simulink subsystem "PvtSubSys_PLAN_AP"  (R2020b)
settings: Solver=VariableStepAuto  StartTime=0.0  StopTime=10.0  RelTol=1e-3
undefined symbols (not defined in the file or in its folder): C_LongCtrl_0_Single, C_LongCtrl_0_Uint8, C_LongCtrl_Mph2Kph, magnitude, P_LongCtrl_accelTargAbsThrd, P_LongCtrl_AddVelAccelChange, P_LongCtrl_AddVelAccelThrd, P_LongCtrl_AddVelDistDesThrd, P_LongCtrl_AddVelEnable, P_LongCtrl_AddVelRefMsThrd, P_LongCtrl_ALaLowerChar, P_LongCtrl_ALaUpperCharEco, P_LongCtrl_ALaUpperCharNormal, P_LongCtrl_ALaUpperCharSport, P_LongCtrl_ALCAccLimitByDangerXAxis, P_LongCtrl_ALCAccLimitByDangerYAxis, P_LongCtrl_ALvAcceleLowerChar, P_LongCtrl_ALvAcceleUpperCharEco, P_LongCtrl_ALvAcceleUpperCharNormal, P_LongCtrl_ALvAcceleUpperCharSport, P_LongCtrl_CCaccelCCNeg2PosJerk, P_LongCtrl_CCaccelCCPosJerk, P_LongCtrl_CCaccelLowerIsLaneChange, P_LongCtrl_CCaccelMaxLCActive, P_LongCtrl_CCaccelMinECOAL, P_LongCtrl_CCaccelMinFastDecel, P_LongCtrl_CCaccelMinNoFastDecel, P_LongCtrl_CCaccelMinNormAL, P_LongCtrl_CCaccelMinSportAL, P_LongCtrl_CCaccelUpperCC, P_LongCtrl_CCaccelUpperCCSafeStop, P_LongCtrl_CCaMinNegAcceleLowerBand, P_LongCtrl_CCaMinNegAcceleUpperBand, P_LongCtrl_CCaMinPosAcceleLowerBand, P_LongCtrl_CCaMinPosAcceleUpperBand, P_LongCtrl_CCbECO, P_LongCtrl_CCbNorm, P_LongCtrl_CCbSport, P_LongCtrl_CCcoefESPSpd2IPSpd1, P_LongCtrl_CCcoefESPSpd2IPSpd2, P_LongCtrl_CCdecelCCJerk, P_LongCtrl_CCdecelCCJerkNegVLCInternalAcc, P_LongCtrl_CCfacNegAcceleLowerBand, P_LongCtrl_CCfacNegAcceleUpperBand, P_LongCtrl_CCfacPosAcceleLowerBand, P_LongCtrl_CCfacPosAcceleUpperBand, P_LongCtrl_CCkECO, P_LongCtrl_CCkNorm, P_LongCtrl_CCkSport, P_LongCtrl_CCLCIncSetSpdAdd, P_LongCtrl_CCLCIncSetSpdAddCntStartValue, P_LongCtrl_CCResumeDelayDeltaVel, P_LongCtrl_CCtAcceleTimeNeg, P_LongCtrl_CCtAcceleTimeNegCorrXAxis, P_LongCtrl_CCtAcceleTimeNegCorrYAxis, P_LongCtrl_CCtAcceleTimePos, P_LongCtrl_CCtAcceleTimePosCorrXAxis, P_LongCtrl_CCtAcceleTimePosCorrYAxis, P_LongCtrl_CCtStepVelPlan, P_LongCtrl_CCtTotVelPlan ... (+150)
libraries: simulink x62, TrueDurationTime x1
(part 2 of 7)

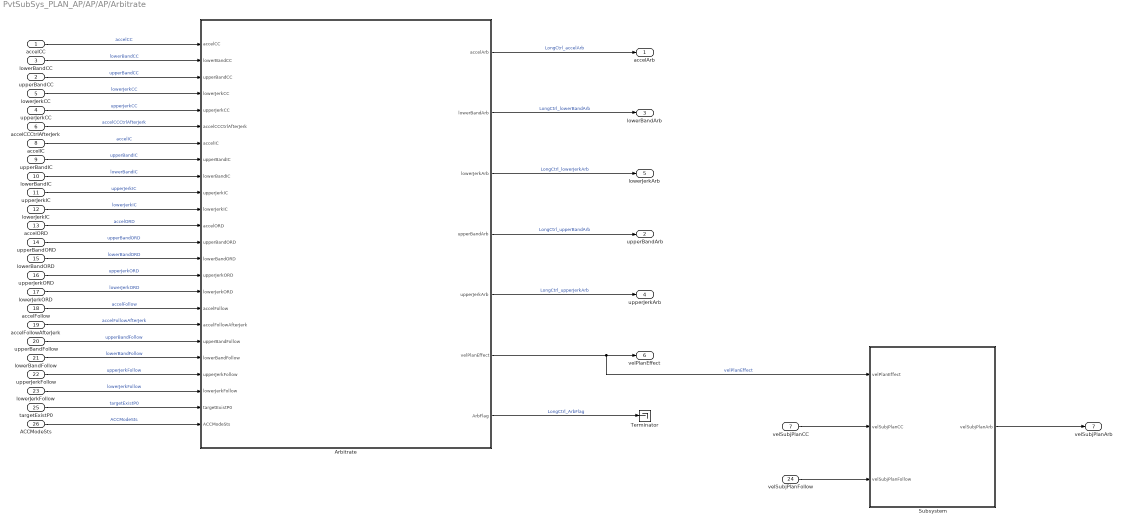
== system PvtSubSys_PLAN_AP/AP/AP/Arbitrate ==
  accelCC : Inport  OutDataTypeStr=single
  upperBandCC : Inport  Port=2  OutDataTypeStr=single
  lowerBandCC : Inport  Port=3  OutDataTypeStr=single
  upperJerkCC : Inport  Port=4  OutDataTypeStr=single
  lowerJerkCC : Inport  Port=5  OutDataTypeStr=single
  accelCCCtrlAfterJerk : Inport  Port=6  OutDataTypeStr=single
  velSubjPlanCC : Inport  Port=7
  accelIC : Inport  Port=8  OutDataTypeStr=single
  upperBandIC : Inport  Port=9  OutDataTypeStr=single
  lowerBandIC : Inport  Port=10  OutDataTypeStr=single
  upperJerkIC : Inport  Port=11  OutDataTypeStr=single
  lowerJerkIC : Inport  Port=12  OutDataTypeStr=single
  accelORD : Inport  Port=13
  upperBandORD : Inport  Port=14
  lowerBandORD : Inport  Port=15
  upperJerkORD : Inport  Port=16
  lowerJerkORD : Inport  Port=17
  accelFollow : Inport  Port=18  OutDataTypeStr=single
  accelFollowAfterJerk : Inport  Port=19
  upperBandFollow : Inport  Port=20  OutDataTypeStr=single
  lowerBandFollow : Inport  Port=21  OutDataTypeStr=single
  upperJerkFollow : Inport  Port=22  OutDataTypeStr=single
  lowerJerkFollow : Inport  Port=23  OutDataTypeStr=single
  velSubjPlanFollow : Inport  Port=24
  targetExistP0 : Inport  Port=25  OutDataTypeStr=boolean
  ACCModeSts : Inport  Port=26  OutDataTypeStr=uint8
  Arbitrate : Stateflow chart  TreatAsAtomicUnit=on
  Subsystem : Subsystem
  Terminator : Terminator
  accelArb : Outport  OutDataTypeStr=single
  " upperBandArb" : Outport  Port=2  OutDataTypeStr=single
  " lowerBandArb" : Outport  Port=3  OutDataTypeStr=single
  " upperJerkArb" : Outport  Port=4  OutDataTypeStr=single
  lowerJerkArb : Outport  Port=5  OutDataTypeStr=single
  velPlanEffect : Outport  Port=6  OutDataTypeStr=uint8
  velSubjPlanArb : Outport  Port=7  OutDataTypeStr=single
  wires:
  Arbitrate/7(ArbFlag) -> Terminator/1  "LongCtrl_ArbFlag"
  lowerJerkIC/1 -> Arbitrate/11(lowerJerkIC)  "lowerJerkIC"
  upperJerkIC/1 -> Arbitrate/10(upperJerkIC)  "upperJerkIC"
  lowerBandIC/1 -> Arbitrate/9(lowerBandIC)  "lowerBandIC"
  upperBandIC/1 -> Arbitrate/8(upperBandIC)  "upperBandIC"
  accelIC/1 -> Arbitrate/7(accelIC)  "accelIC"
  accelCCCtrlAfterJerk/1 -> Arbitrate/6(accelCCCtrlAfterJerk)  "accelCCCtrlAfterJerk"
  ACCModeSts/1 -> Arbitrate/24(ACCModeSts)  "ACCModeSts"
  Arbitrate/3(lowerJerkArb) -> lowerJerkArb/1  "LongCtrl_lowerJerkArb"
  Arbitrate/5(upperJerkArb) -> " upperJerkArb"/1  "LongCtrl_upperJerkArb"
  Arbitrate/2(lowerBandArb) -> " lowerBandArb"/1  "LongCtrl_lowerBandArb"
  Arbitrate/4(upperBandArb) -> " upperBandArb"/1  "LongCtrl_upperBandArb"
  Arbitrate/1(accelArb) -> accelArb/1  "LongCtrl_accelArb"
  targetExistP0/1 -> Arbitrate/23(targetExistP0)  "targetExistP0"
  lowerJerkFollow/1 -> Arbitrate/22(lowerJerkFollow)  "lowerJerkFollow"
  upperJerkFollow/1 -> Arbitrate/21(upperJerkFollow)  "upperJerkFollow"
  lowerBandFollow/1 -> Arbitrate/20(lowerBandFollow)  "lowerBandFollow"
  upperBandFollow/1 -> Arbitrate/19(upperBandFollow)  "upperBandFollow"
  accelFollow/1 -> Arbitrate/17(accelFollow)  "accelFollow"
  lowerJerkCC/1 -> Arbitrate/4(lowerJerkCC)  "lowerJerkCC"
  upperJerkCC/1 -> Arbitrate/5(upperJerkCC)  "upperJerkCC"
  lowerBandCC/1 -> Arbitrate/2(lowerBandCC)  "lowerBandCC"
  upperBandCC/1 -> Arbitrate/3(upperBandCC)  "upperBandCC"
  accelCC/1 -> Arbitrate/1(accelCC)  "accelCC"
  accelFollowAfterJerk/1 -> Arbitrate/18(accelFollowAfterJerk)  "accelFollowAfterJerk"
  accelORD/1 -> Arbitrate/12(accelORD)  "accelORD"
  upperBandORD/1 -> Arbitrate/13(upperBandORD)  "upperBandORD"
  lowerJerkORD/1 -> Arbitrate/16(lowerJerkORD)  "lowerJerkORD"
  upperJerkORD/1 -> Arbitrate/15(upperJerkORD)  "upperJerkORD"
  lowerBandORD/1 -> Arbitrate/14(lowerBandORD)  "lowerBandORD"
  Arbitrate/6(velPlanEffect) -> Subsystem/1(velPlanEffect), velPlanEffect/1  "velPlanEffect"
  velSubjPlanCC/1 -> Subsystem/2(velSubjPlanCC)
  velSubjPlanFollow/1 -> Subsystem/3(velSubjPlanFollow)
  Subsystem/1(velSubjPlanArb) -> velSubjPlanArb/1

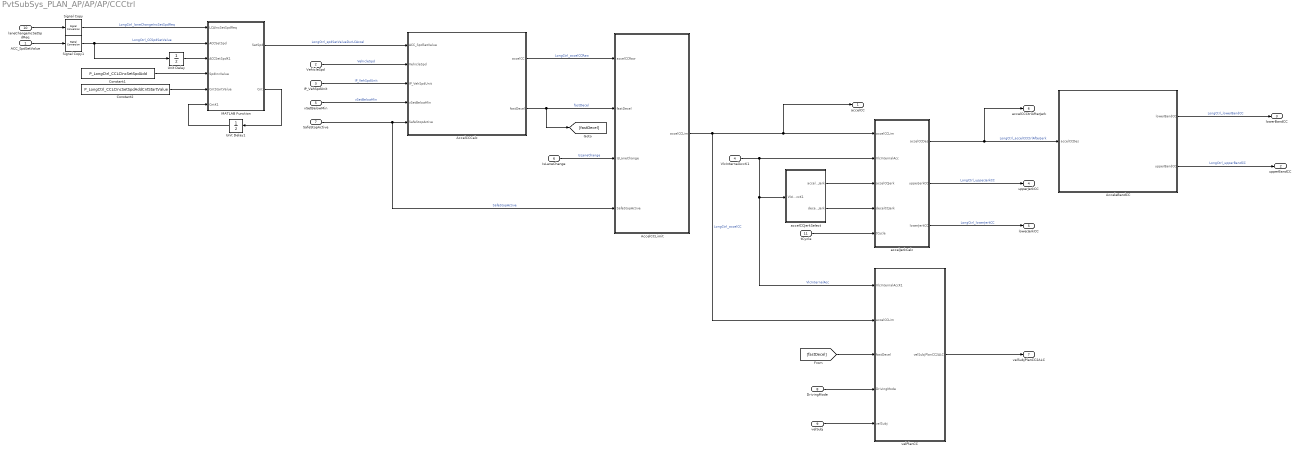
== system PvtSubSys_PLAN_AP/AP/AP/CCCtrl ==
  ACC_SpdSetValue : Inport  OutDataTypeStr=single
  VehicleSpd : Inport  Port=2  OutDataTypeStr=single
  IP_VehSpdUnit : Inport  Port=3  OutDataTypeStr=uint8
  VlcInternalAccK1 : Inport  Port=4  OutDataTypeStr=single
  vSetBelowMin : Inport  Port=5  OutDataTypeStr=boolean
  IsLaneChange : Inport  Port=6  OutDataTypeStr=boolean
  SafeStopActive : Inport  Port=7  OutDataTypeStr=boolean
  DrivingMode : Inport  Port=8
  velSubj : Inport  Port=9
  laneChangeIncSetSpdReq : Inport  Port=10
  tCycle : Inport  Port=11  OutDataTypeStr=single
  AccelCCCalc : Stateflow chart  TreatAsAtomicUnit=on
  AccelCCLimit : Subsystem
  AcceleBandCC : Stateflow chart  TreatAsAtomicUnit=on
  Constant1 : Constant  Value=P_LongCtrl_CCLCIncSetSpdAdd
  Constant2 : Constant  Value=P_LongCtrl_CCLCIncSetSpdAddCntStartValue
  MATLAB Function : MATLAB Function  TreatAsAtomicUnit=on
  Signal Copy : SignalConversion  OverrideOpt=off
  Signal Copy1 : SignalConversion  OverrideOpt=off
  Unit Delay : UnitDelay  SampleTime=-1  HasFrameUpgradeWarning=on
  Unit Delay1 : UnitDelay  SampleTime=-1  HasFrameUpgradeWarning=on
  accelCCJerkSelect : Subsystem
  accelJerkCalc : Subsystem
  velPlanCC : Subsystem
  accelCC : Outport  OutDataTypeStr=single
  upperBandCC : Outport  Port=2  OutDataTypeStr=single
  lowerBandCC : Outport  Port=3  OutDataTypeStr=single
  upperJerkCC : Outport  Port=4  OutDataTypeStr=single
  lowerJerkCC : Outport  Port=5  OutDataTypeStr=single
  accelCCCtrlAfterJerk : Outport  Port=6  OutDataTypeStr=single
  velSubjPlanCC2ALC : Outport  Port=7  OutDataTypeStr=single
  wires:
  ACC_SpdSetValue/1 -> Signal Copy1/1
  Signal Copy1/1 -> MATLAB Function/2(ACCSetSpd), Unit Delay/1  "LongCtrl_CCSpdSetValue"
  Signal Copy/1 -> MATLAB Function/1(LCAIncSetSpdReq)  "LongCtrl_laneChangeIncSetSpdReq"
  laneChangeIncSetSpdReq/1 -> Signal Copy/1
  SafeStopActive/1 -> AccelCCCalc/5(SafeStopActive), AccelCCLimit/4(SafeStopActive)  "SafeStopActive"
  IsLaneChange/1 -> AccelCCLimit/3(IsLaneChange)  "IsLaneChange"
  vSetBelowMin/1 -> AccelCCCalc/4(vSetBelowMin)  "vSetBelowMin"
  tCycle/1 -> accelJerkCalc/5(tCycle)
  accelCCJerkSelect/2(decelCCJerk) -> accelJerkCalc/4(decelCCJerk)
  AccelCCCalc/2(fastDecel) -> [fastDecel], AccelCCLimit/2(fastDecel)  "fastDecel"
  AccelCCCalc/1(accelCC) -> AccelCCLimit/1(accelCCRaw)  "LongCtrl_accelCCRaw"
  AccelCCLimit/1(accelCCLim) -> velPlanCC/2(accelCCLim), accelJerkCalc/1(accelCCLim), accelCC/1  "LongCtrl_accelCC"
  accelCCJerkSelect/1(accelCCJerk) -> accelJerkCalc/3(accelCCJerk)
  accelJerkCalc/3(lowerJerkCC) -> lowerJerkCC/1  "LongCtrl_lowerJerkCC"
  accelJerkCalc/2(upperJerkCC) -> upperJerkCC/1  "LongCtrl_upperJerkCC"
  AcceleBandCC/1(lowerBandCC) -> lowerBandCC/1  "LongCtrl_lowerBandCC"
  AcceleBandCC/2(upperBandCC) -> upperBandCC/1  "LongCtrl_upperBandCC"
  VlcInternalAccK1/1 -> accelJerkCalc/2(VlcInternalAcc), velPlanCC/1(VlcInternalAccK1), accelCCJerkSelect/1(VlcInternalAccK1)  "VlcInternalAcc"
  accelJerkCalc/1(accelCCDes) -> AcceleBandCC/1(accelCCDes), accelCCCtrlAfterJerk/1  "LongCtrl_accelCCCtrlAfterJerk"
  IP_VehSpdUnit/1 -> AccelCCCalc/3(IP_VehSpdUnit)  "IP_VehSpdUnit"
  VehicleSpd/1 -> AccelCCCalc/2(VehicleSpd)  "VehicleSpd"
  [fastDecel] -> velPlanCC/3(fastDecel)
  DrivingMode/1 -> velPlanCC/4(DrivingMode)
  velSubj/1 -> velPlanCC/5(velSubj)
  velPlanCC/1(velSubjPlanCC2ALC) -> velSubjPlanCC2ALC/1
  MATLAB Function/2(Cnt) -> Unit Delay1/1
  MATLAB Function/1(SetSpd) -> AccelCCCalc/1(ACC_SpdSetValue)  "LongCtrl_spdSetValueDurLCAccel"
  Unit Delay1/1 -> MATLAB Function/6(CntK1)
  Constant2/1 -> MATLAB Function/5(CntStartValue)
  Unit Delay/1 -> MATLAB Function/3(ACCSetSpdK1)
  Constant1/1 -> MATLAB Function/4(SpdIncValue)

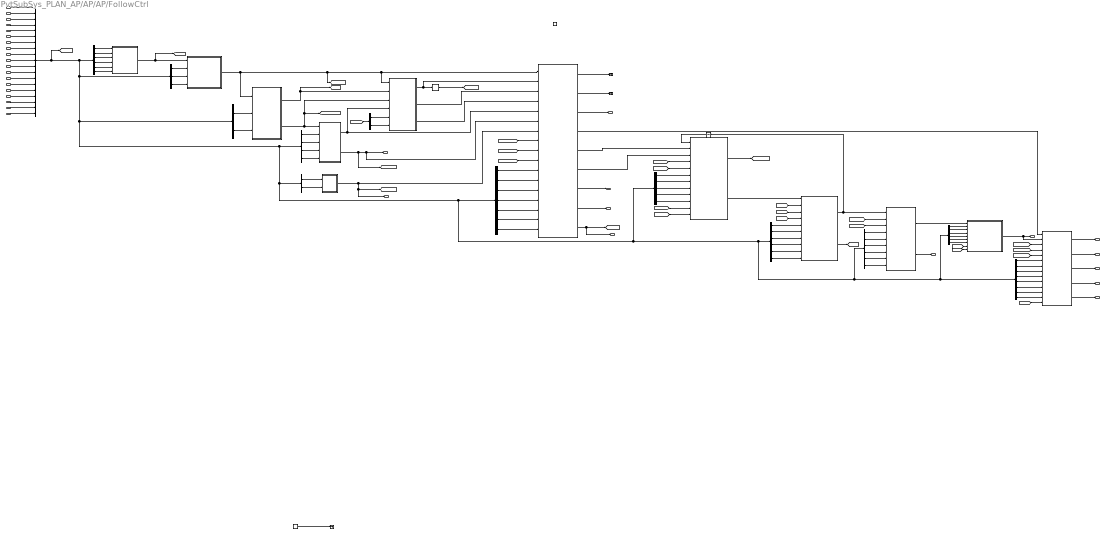
== system PvtSubSys_PLAN_AP/AP/AP/FollowCtrl ==
  VlcInternalAccK20 : Inport
  velSubj : Inport  Port=2
  VlcInternalAccK1 : Inport  Port=3
  distTargRel : Inport  Port=4
  velTargRel : Inport  Port=5
  accelTargAbsP0 : Inport  Port=6
  timeGap : Inport  Port=7
  ACCModeSts : Inport  Port=8  OutDataTypeStr=uint8
  IDP0 : Inport  Port=9  OutDataTypeStr=uint8
  IDP2 : Inport  Port=10  OutDataTypeStr=uint8
  IDP3 : Inport  Port=11  OutDataTypeStr=uint8
  accelTargAbsP2 : Inport  Port=12
  accelTargAbsP3 : Inport  Port=13
  dangerLevel : Inport  Port=14
  laneChangeEnable : Inport  Port=15
  axvRoadSlopeMs2 : Inport  Port=16
  ObjMovingStateP0 : Inport  Port=17
  tCycle : Inport  Port=18
  DrvOFF_Req : Inport  Port=19
  Enable : EnablePort
  AccelSupression : Subsystem
  AccelTargAbsEnableJudge : Subsystem
  AccelTargFilter : Subsystem
  Bus Creator : BusCreator  Inputs=19
  Bus Selector : BusSelector  OutputSignals=IDP0,IDP2,IDP3,accelTargAbsP0,accelTargAbsP2,accelTargAbsP3
  Bus Selector1 : BusSelector  OutputSignals=distTargRel,tCycle,IDP0
  Bus Selector10 : BusSelector  OutputSignals=velSubj,velTargRel,IDP0,distTargRel,LongCtrl_ALC_dangerLevel,LongCtrl_ALC_laneChangeEnable
  Bus Selector11 : BusSelector  OutputSignals=axvRoadSlopeMs2,velSubj,velTargRel,distTargRel,ACCModeSts,tCycle
  Bus Selector2 : BusSelector  OutputSignals=velTargRel,velSubj
  Bus Selector3 : BusSelector  OutputSignals=timeGap,distTargRel,velTargRel,velSubj
  Bus Selector4 : BusSelector  OutputSignals=velTargRel,distTargRel
  Bus Selector5 : BusSelector  OutputSignals=distTargRel,velSubj
  Bus Selector6 : BusSelector  OutputSignals=distTargRel,velSubj,VlcInternalAccK20,velTargRel,IDP0,ACCModeSts,tCycle
  Bus Selector7 : BusSelector  OutputSignals=velSubj,IDP0,distTargRel,ACCModeSts,velTargRel
  Bus Selector8 : BusSelector  OutputSignals=distTargRel,velSubj,ACCModeSts,DrvOFF_Req,axvRoadSlopeMs2,ObjMovingStateP0
  Bus Selector9 : BusSelector  OutputSignals=VlcInternalAccK1,distTargRel,velSubj,ACCModeSts,tCycle,velTargRel,IDP0,axvRoadSlopeMs2
  Counter Limited : simulink/Sources/Counter Limited  uplimit=15  tsamp=-1
  DecelToStopCtrl : Subsystem
  DistDesCalc : Subsystem
  DistRelPlanTerminateCalc : Subsystem
  FollowBandJerkCalc : Subsystem
  Permute Dimensions1 : PermuteDimensions
  PlausibilityCheck : Subsystem
  SlopeStartupAssist : Subsystem
  TTC : Subsystem
  Terminator : Terminator
  Terminator1 : Terminator
  Terminator3 : Terminator
  Unit Delay : UnitDelay  SampleTime=-1  HasFrameUpgradeWarning=on
  VelPlan : Subsystem
  VelTargPlanTerminateCalc : Subsystem
  accelFollow : Outport  OutDataTypeStr=single
  upperBandFollow : Outport  Port=2  OutDataTypeStr=single
  lowerBandFollow : Outport  Port=3  OutDataTypeStr=single
  upperJerkFollow : Outport  Port=4  OutDataTypeStr=single
  lowerJerkFollow : Outport  Port=5  OutDataTypeStr=single
  distRelPlanMin : Outport  Port=6  OutDataTypeStr=single
  distRelDesDistRelPlanNumMin : Outport  Port=7  OutDataTypeStr=single
  distDesCur : Outport  Port=8  OutDataTypeStr=single
  tStartDecel : Outport  Port=9  OutDataTypeStr=single
  accelFollowAfterJerk : Outport  Port=10  OutDataTypeStr=single
  velSubjPlanFollow : Outport  Port=11  OutDataTypeStr=single
  ttc : Outport  Port=12
  accelSubjPlanOpt : Outport  Port=13
  wires:
  Bus Selector8/6 -> DecelToStopCtrl/10(ObjMovingStateP0)  "<ObjMovingStateP0>"
  ObjMovingStateP0/1 -> Bus Creator/19  "ObjMovingStateP0"
  [accelTargAbsFilt] -> FollowBandJerkCalc/14(accelTargAbsFilt)
  Bus Selector6/7 -> VelPlan/17(tCycle)  "<tCycle>"
  Bus Selector6/6 -> VelPlan/16(ACCModeSts)  "<ACCModeSts>"
  Counter Limited/1 -> Terminator3/1  "LongCtrl_Follow_Counter"
  Bus Selector10/4 -> AccelSupression/7(distTargRel)  "<distTargRel>"
  Bus Selector10/1 -> AccelSupression/4(velSubj)  "<velSubj>"
  Bus Selector10/6 -> AccelSupression/9(laneChangeEnable)  "<LongCtrl_ALC_laneChangeEnable>"
  Bus Selector10/2 -> AccelSupression/5(velTargRel)  "<velTargRel>"
  Bus Selector10/5 -> AccelSupression/8(dangerLevel)  "<LongCtrl_ALC_dangerLevel>"
  Bus Selector10/3 -> AccelSupression/6(IDP0)  "<IDP0>"
  laneChangeEnable/1 -> Bus Creator/17  "LongCtrl_ALC_laneChangeEnable"
  dangerLevel/1 -> Bus Creator/16  "LongCtrl_ALC_dangerLevel"
  [accelTargAbsEnable] -> AccelSupression/3(accelTargAbsEnable)
  [accelSubjPlanOpt] -> AccelSupression/2(accelSubjPlanOpt)  "accelSubjPlanOpt"
  VelPlan/9(accelSubjPlanOpt) -> accelSubjPlanOpt/1, [accelSubjPlanOpt]  "accelSubjPlanOpt"
  AccelSupression/2(tStartDecel) -> tStartDecel/1  "tStartDecel"
  SlopeStartupAssist/1(accelFollowSlopeAssist) -> FollowBandJerkCalc/2(accelFollow), accelFollow/1  "LongCtrl_accelFollow"
  Bus Selector/1 -> AccelTargFilter/1(IDP0)  "<IDP0>"
  Bus Selector/2 -> AccelTargFilter/2(IDP2)  "<IDP2>"
  Bus Selector/6 -> AccelTargFilter/6(accelTargAbsP3)  "<accelTargAbsP3>"
  Bus Selector/3 -> AccelTargFilter/3(IDP3)  "<IDP3>"
  Bus Selector/5 -> AccelTargFilter/5(accelTargAbsP2)  "<accelTargAbsP2>"
  Bus Selector/4 -> AccelTargFilter/4(accelTargAbsP0)  "<accelTargAbsP0>"
  IDP3/1 -> Bus Creator/13  "IDP3"
  IDP2/1 -> Bus Creator/12  "IDP2"
  accelTargAbsP2/1 -> Bus Creator/14  "accelTargAbsP2"
  accelTargAbsP3/1 -> Bus Creator/15  "accelTargAbsP3"
  Bus Selector9/6 -> FollowBandJerkCalc/11(velTargRel)  "<velTargRel>"
  Bus Selector9/5 -> FollowBandJerkCalc/10(tCycle)  "<tCycle>"
  Bus Selector9/1 -> FollowBandJerkCalc/6(VlcInternalAccK1)  "<VlcInternalAccK1>"
  Bus Selector9/4 -> FollowBandJerkCalc/9(ACCModeSts)  "<ACCModeSts>"
  Bus Selector9/2 -> FollowBandJerkCalc/7(distTargRel)  "<distTargRel>"
  Bus Selector9/3 -> FollowBandJerkCalc/8(velSubj)  "<velSubj>"
  [accelTargAbsFilt] -> DecelToStopCtrl/4(accelTargAbsFilt)
  Bus Selector8/4 -> DecelToStopCtrl/8(DrvOFF_Req)  "<DrvOFF_Req>"
  Bus Selector8/3 -> DecelToStopCtrl/7(ACCModeSts)  "<ACCModeSts>"
  Bus Selector8/2 -> DecelToStopCtrl/6(velSubj)  "<velSubj>"
  Bus Selector8/1 -> DecelToStopCtrl/5(distTargRel)  "<distTargRel>"
  Bus Selector7/4 -> PlausibilityCheck/9(ACCMode)  "<ACCModeSts>"
  Bus Selector7/3 -> PlausibilityCheck/8(distTargRel)  "<distTargRel>"
  Bus Selector7/2 -> PlausibilityCheck/7(IDP0)  "<IDP0>"
  Bus Selector7/1 -> PlausibilityCheck/6(velSubj)  "<velSubj>"
  Bus Selector6/1 -> VelPlan/11(distTargRel)  "<distTargRel>"
  Bus Selector6/2 -> VelPlan/12(velSubj)  "<velSubj>"
  Bus Selector6/5 -> VelPlan/15(IDP0)  "<IDP0>"
  Bus Selector6/3 -> VelPlan/13(VlcInternalAccK20)  "<VlcInternalAccK20>"
  Bus Selector6/4 -> VelPlan/14(velTargRel)  "<velTargRel>"
  Bus Selector5/1 -> DistRelPlanTerminateCalc/5(distTargRel)  "<distTargRel>"
  Bus Selector5/2 -> DistRelPlanTerminateCalc/6(velSubj)  "<velSubj>"
  [InSingal] -> Bus Selector5/1
  Bus Selector4/1 -> TTC/1(velTargRel)  "<velTargRel>"
  Bus Selector4/2 -> TTC/2(distTargRel)  "<distTargRel>"
  Bus Selector3/1 -> DistDesCalc/2(timeGap)  "<timeGap>"
  Bus Selector3/2 -> DistDesCalc/3(distTargRel)  "<distTargRel>"
  Bus Selector3/3 -> DistDesCalc/4(velTargRel)  "<velTargRel>"
  Bus Selector3/4 -> DistDesCalc/5(velSubj)  "<velSubj>"
  Bus Selector2/2 -> VelTargPlanTerminateCalc/3(velSubj)  "<velSubj>"
  Bus Selector2/1 -> VelTargPlanTerminateCalc/2(velTargRel)  "<velTargRel>"
  Bus Selector1/2 -> AccelTargAbsEnableJudge/3(tCycle)  "<tCycle>"
  Bus Selector1/1 -> AccelTargAbsEnableJudge/2(distTargRel)  "<distTargRel>"
  Bus Creator/1 -> Bus Selector/1, Bus Selector2/1, Bus Selector3/1, Bus Selector4/1, Bus Selector6/1, Bus Selector8/1, Bus Selector9/1, Bus Selector11/1, Bus Selector10/1, Bus Selector7/1, Bus Selector1/1, [InSingal]
  DrvOFF_Req/1 -> Bus Creator/11  "DrvOFF_Req"
  tCycle/1 -> Bus Creator/10  "tCycle"
  IDP0/1 -> Bus Creator/9  "IDP0"
  ACCModeSts/1 -> Bus Creator/8  "ACCModeSts"
  timeGap/1 -> Bus Creator/7  "timeGap"
  accelTargAbsP0/1 -> Bus Creator/6  "accelTargAbsP0"
  velTargRel/1 -> Bus Creator/5  "velTargRel"
  distTargRel/1 -> Bus Creator/4  "distTargRel"
  VlcInternalAccK20/1 -> Bus Creator/1  "VlcInternalAccK20"
  VlcInternalAccK1/1 -> Bus Creator/3  "VlcInternalAccK1"
  velSubj/1 -> Bus Creator/2  "velSubj"
  Unit Delay/1 -> PlausibilityCheck/1(FollowAcceleK1)
  [ttc] -> FollowBandJerkCalc/4(ttc)
  [PlauCheckEnable] -> FollowBandJerkCalc/3(PlauCheckEnable)
  PlausibilityCheck/1(PlauCheckEnable) -> [PlauCheckEnable]
  DecelToStopCtrl/1(accelFollowAfterDecelToStop) -> AccelSupression/1(accelFollow), Unit Delay/1
  VelPlan/6(num1) -> PlausibilityCheck/3(num)
  [distRelPlanTerminate] -> PlausibilityCheck/5(distRelPlanTerminate)
  [velTargAbs] -> PlausibilityCheck/4(velTargAbs)
  VelPlan/5(accelSubjPlan) -> PlausibilityCheck/2(accelSubjPlan)  "LongCtrl_accelSubjDesCorr"
  TTC/1(ttc) -> VelPlan/7(ttc), [ttc], ttc/1  "ttc"
  VelPlan/4(Gap2) -> FollowBandJerkCalc/1(Gap)
  VelPlan/8(distRelDesDistRelPlanNumMin) -> distRelDesDistRelPlanNumMin/1
  VelPlan/7(distRelPlanMin) -> distRelPlanMin/1
  [velTargAbs] -> DecelToStopCtrl/3(velTargAbs)
  [accelTargAbsFilt] -> VelPlan/10(accelTargAbsFilt)
  DistRelPlanTerminateCalc/3(distTargPlan) -> VelPlan/4(distTargPlan)
  DistRelPlanTerminateCalc/2(tTargStop) -> VelPlan/3(tTargStop)
  DistDesCalc/2(distDesCur) -> distDesCur/1, VelPlan/6(distDesCur), [distDesCur]  "LongCtrl_distDesCur"
  FollowBandJerkCalc/4(lowerJerkFollow) -> lowerJerkFollow/1
  FollowBandJerkCalc/3(" upperJerkFollow") -> upperJerkFollow/1
  [distDesCur] -> DecelToStopCtrl/2(distDesCur)
  Permute Dimensions1/1 -> [distRelPlanTerminate]  "LongCtrl_distRelPlanTerminate"
  PlausibilityCheck/2(followAcceleStandstillOverride) -> DecelToStopCtrl/1(accelFollow)  "LongCtrl_FollowAcceleStandstillOverride"
  [velTargAbs] -> VelPlan/9(velTargAbs)
  [velTargAbsPlanTerminate] -> VelPlan/8(velTargAbsPlanTerminate)
  VelPlan/1(distRelPlan) -> Terminator/1  "LongCtrl_distRelPlanOpt"
  VelPlan/3(velSubjPlan) -> velSubjPlanFollow/1  "LongCtrl_velSubjPlanOpt"
  VelPlan/2(velPlanRel) -> Terminator1/1  "LongCtrl_velPlanRelOpt"
  VelTargPlanTerminateCalc/2(velTargAbsPlanTerminate) -> [velTargAbsPlanTerminate], DistRelPlanTerminateCalc/3(velTargAbsPlanTerminate), DistDesCalc/1(velTargAbsPlanTerminate)
  VelTargPlanTerminateCalc/1(velTargAbs) -> [velTargAbs], DistRelPlanTerminateCalc/2(velTargAbs)
  DistRelPlanTerminateCalc/1(distRelPlanTerminate) -> VelPlan/2(distRelPlanTerminate), Permute Dimensions1/1
  DistDesCalc/1(distDesPlanCorr) -> DistRelPlanTerminateCalc/4(distDesPlanCorr), VelPlan/5(distDesPlanCorr)  "LongCtrl_distDesPlanCorr"
  AccelTargFilter/1(accelTargAbsFilt) -> [accelTargAbsFilt], AccelTargAbsEnableJudge/1(accelTargAbsFilt)  "LongCtrl_accelTargAbsFilt"
  AccelTargAbsEnableJudge/1(accelTargAbsEnable) -> VelTargPlanTerminateCalc/1(accelTargAbsEnable), VelPlan/1(accelTargAbs), DistRelPlanTerminateCalc/1(accelTargAbsEnable), [accelTargAbsEnable]  "LongCtrl_accelTargAbsEnable"
  FollowBandJerkCalc/1(upperBandFollow) -> upperBandFollow/1  "LongCtrl_upperBandFollow"
  FollowBandJerkCalc/2(lowerBandFollow) -> lowerBandFollow/1  "LongCtrl_lowerBandFollow"
  AccelSupression/1(accelFollowAfterLaneChangeSupress) -> SlopeStartupAssist/1(accelFollowAfterLaneChangeSupress)
  axvRoadSlopeMs2/1 -> Bus Creator/18  "axvRoadSlopeMs2"
  Bus Selector11/1 -> SlopeStartupAssist/2(axvRoadSlopeMs2)  "<axvRoadSlopeMs2>"
  Bus Selector11/2 -> SlopeStartupAssist/3(velSubj)  "<velSubj>"
  FollowBandJerkCalc/5(accelFollowAfterJerk) -> accelFollowAfterJerk/1
  Bus Selector8/5 -> DecelToStopCtrl/9(axvRoadSlopeMs2)  "<axvRoadSlopeMs2>"
  DecelToStopCtrl/2(ForceStop) -> [ForceStop]
  [ForceStop] -> FollowBandJerkCalc/5(ForceStop)
  Bus Selector9/7 -> FollowBandJerkCalc/12(IDP0)  "<IDP0>"
  Bus Selector9/8 -> FollowBandJerkCalc/13(axvRoadSlopeMs2)  "<axvRoadSlopeMs2>"
  Bus Selector1/3 -> AccelTargAbsEnableJudge/4(IDP0)  "<IDP0>"
  [distDesCur] -> PlausibilityCheck/12(distDesCur)
  [accelTargAbsEnable] -> PlausibilityCheck/11(accelTargAbsEnable)
  Bus Selector7/5 -> PlausibilityCheck/10(velTargRel)  "<velTargRel>"
  Bus Selector11/3 -> SlopeStartupAssist/4(velTargRel)  "<velTargRel>"
  Bus Selector11/4 -> SlopeStartupAssist/5(distTargRel)  "<distTargRel>"
  [distDesCur] -> SlopeStartupAssist/8(distDesCur)
  [velTargAbs] -> SlopeStartupAssist/9(velTargAbs)
  Bus Selector11/5 -> SlopeStartupAssist/6(ACCModeSts)  "<ACCModeSts>"
  Bus Selector11/6 -> SlopeStartupAssist/7(tCycle)  "<tCycle>"

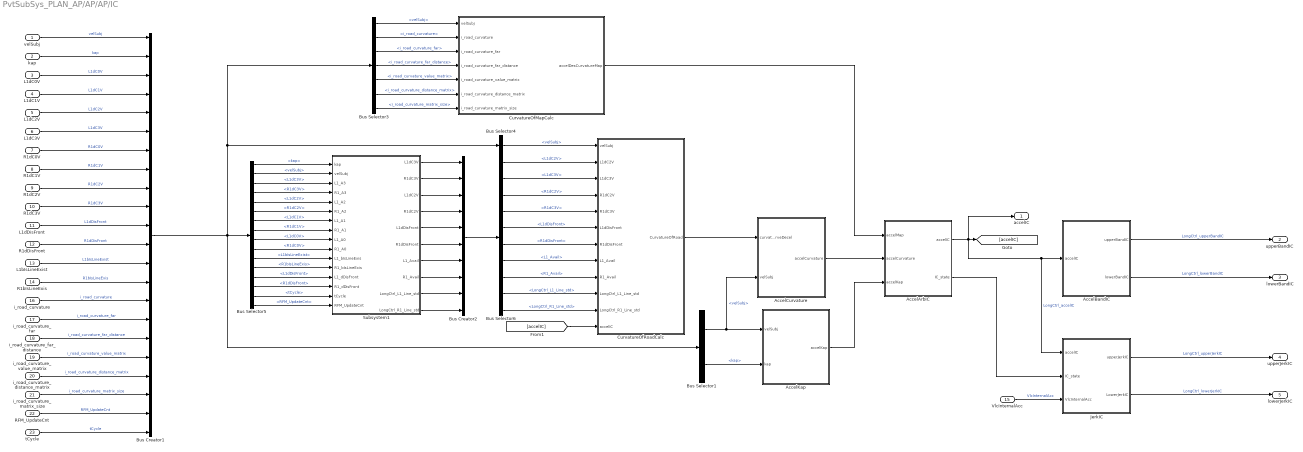
== system PvtSubSys_PLAN_AP/AP/AP/IC ==
  velSubj : Inport
  kap : Inport  Port=2
  L1dC0V : Inport  Port=3
  L1dC1V : Inport  Port=4
  L1dC2V : Inport  Port=5
  L1dC3V : Inport  Port=6
  R1dC0V : Inport  Port=7
  R1dC1V : Inport  Port=8
  R1dC2V : Inport  Port=9
  R1dC3V : Inport  Port=10
  L1dDisFront : Inport  Port=11
  R1dDisFront : Inport  Port=12
  L1bIsLineExist : Inport  Port=13
  R1bIsLineExis : Inport  Port=14
  VlcInternalAcc : Inport  Port=15
  i_road_curvature : Inport  Port=16
  i_road_curvature_far : Inport  Port=17
  i_road_curvature_far_distance : Inport  Port=18
  i_road_curvature_value_matrix : Inport  Port=19
  i_road_curvature_distance_matrix : Inport  Port=20
  i_road_curvature_matrix_size : Inport  Port=21
  RFM_UpdateCnt : Inport  Port=22
  tCycle : Inport  Port=23
  AccelArbIC : Subsystem  Description=Acceleration Intelligence Curve Arbitrate
  AccelBandIC : Subsystem  Description=Acceleration Intelligence Curve Arbitrate
  AccelCurvature : Subsystem
  AccelKap : Subsystem
  Bus Creator1 : BusCreator  Inputs=22
  Bus Creator2 : BusCreator  Inputs=10
  Bus Selector1 : BusSelector  OutputSignals=velSubj,kap
  Bus Selector3 : BusSelector  OutputSignals=velSubj,i_road_curvature,i_road_curvature_far,i_road_curvature_far_distance,i_road_curvature_value_matrix,i_road_curvature_distance_matrix,i_road_curvature_matrix_size
  Bus Selector4 : BusSelector  OutputSignals=velSubj
  Bus Selector5 : BusSelector  OutputSignals=kap,velSubj,L1dC3V,R1dC3V,L1dC2V,R1dC2V,L1dC1V,R1dC1V,L1dC0V,R1dC0V,L1bIsLineExist,R1bIsLineExis,L1dDisFront,R1dDisFront,tCycle,RFM_UpdateCnt
  Bus Selector6 : BusSelector  OutputSignals=L1dC2V,L1dC3V,R1dC2V,R1dC3V,L1dDisFront,R1dDisFront,L1_Avail,R1_Avail,LongCtrl_L1_Line_std,LongCtrl_R1_Line_std
  CurvatureOfMapCalc : Subsystem
  CurvatureOfRoadCalc : Subsystem
  JerkIC : Subsystem  Description=Acceleration Intelligence Curve Arbitrate
  Subsystem1 : Subsystem
  accelIC : Outport  OutDataTypeStr=single
  upperBandIC : Outport  Port=2  OutDataTypeStr=single
  lowerBandIC : Outport  Port=3  OutDataTypeStr=single
  upperJerkIC : Outport  Port=4  OutDataTypeStr=single
  lowerJerkIC : Outport  Port=5  OutDataTypeStr=single
  wires:
  [accelIC] -> CurvatureOfRoadCalc/12(accelIC)
  Bus Selector5/16 -> Subsystem1/16(RFM_UpdateCnt)  "<RFM_UpdateCnt>"
  Bus Selector5/9 -> Subsystem1/9(L1_A0)  "<L1dC0V>"
  Bus Selector5/12 -> Subsystem1/12(R1_bIsLineExis)  "<R1bIsLineExis>"
  Bus Selector6/4 -> CurvatureOfRoadCalc/5(R1dC3V)  "<R1dC3V>"
  Bus Selector6/9 -> CurvatureOfRoadCalc/10(LongCtrl_L1_Line_std)  "<LongCtrl_L1_Line_std>"
  Bus Selector5/6 -> Subsystem1/6(R1_A2)  "<R1dC2V>"
  Bus Selector6/3 -> CurvatureOfRoadCalc/4(R1dC2V)  "<R1dC2V>"
  Bus Selector6/7 -> CurvatureOfRoadCalc/8(L1_Avail)  "<L1_Avail>"
  Subsystem1/6(R1dDisFront) -> Bus Creator2/6
  Bus Selector6/5 -> CurvatureOfRoadCalc/6(L1dDisFront)  "<L1dDisFront>"
  Subsystem1/9(LongCtrl_L1_Line_std) -> Bus Creator2/9
  Bus Selector4/1 -> CurvatureOfRoadCalc/1(velSubj)  "<velSubj>"
  Bus Selector5/10 -> Subsystem1/10(R1_A0)  "<R1dC0V>"
  Subsystem1/7(L1_Avail) -> Bus Creator2/7
  Bus Selector5/1 -> Subsystem1/1(kap)  "<kap>"
  Bus Selector5/8 -> Subsystem1/8(R1_A1)  "<R1dC1V>"
  Bus Selector5/14 -> Subsystem1/14(R1_dDisFront)  "<R1dDisFront>"
  Bus Selector5/7 -> Subsystem1/7(L1_A1)  "<L1dC1V>"
  Bus Selector6/6 -> CurvatureOfRoadCalc/7(R1dDisFront)  "<R1dDisFront>"
  Bus Selector5/11 -> Subsystem1/11(L1_bIsLineExis)  "<L1bIsLineExist>"
  Bus Selector5/15 -> Subsystem1/15(tCycle)  "<tCycle>"
  Bus Selector5/5 -> Subsystem1/5(L1_A2)  "<L1dC2V>"
  Bus Selector5/13 -> Subsystem1/13(L1_dDisFront)  "<L1dDisFront>"
  Bus Selector5/3 -> Subsystem1/3(L1_A3)  "<L1dC3V>"
  Bus Creator2/1 -> Bus Selector6/1
  Bus Selector6/10 -> CurvatureOfRoadCalc/11(LongCtrl_R1_Line_std)  "<LongCtrl_R1_Line_std>"
  Subsystem1/10(LongCtrl_R1_Line_std) -> Bus Creator2/10
  Bus Selector5/4 -> Subsystem1/4(R1_A3)  "<R1dC3V>"
  Subsystem1/4(R1dC2V) -> Bus Creator2/4
  Bus Selector6/1 -> CurvatureOfRoadCalc/2(L1dC2V)  "<L1dC2V>"
  Subsystem1/1(L1dC3V) -> Bus Creator2/1
  Bus Selector6/8 -> CurvatureOfRoadCalc/9(R1_Avail)  "<R1_Avail>"
  Bus Selector6/2 -> CurvatureOfRoadCalc/3(L1dC3V)  "<L1dC3V>"
  Subsystem1/8(R1_Avail) -> Bus Creator2/8
  Bus Creator1/1 -> Bus Selector5/1, Bus Selector4/1, Bus Selector3/1, Bus Selector1/1
  Subsystem1/2(R1dC3V) -> Bus Creator2/2
  Bus Selector5/2 -> Subsystem1/2(velSubj)  "<velSubj>"
  Subsystem1/3(L1dC2V) -> Bus Creator2/3
  Subsystem1/5(L1dDisFront) -> Bus Creator2/5
  i_road_curvature_matrix_size/1 -> Bus Creator1/20  "i_road_curvature_matrix_size"
  i_road_curvature_distance_matrix/1 -> Bus Creator1/19  "i_road_curvature_distance_matrix"
  i_road_curvature_value_matrix/1 -> Bus Creator1/18  "i_road_curvature_value_matrix"
  i_road_curvature_far_distance/1 -> Bus Creator1/17  "i_road_curvature_far_distance"
  i_road_curvature_far/1 -> Bus Creator1/16  "i_road_curvature_far"
  i_road_curvature/1 -> Bus Creator1/15  "i_road_curvature"
  R1dC1V/1 -> Bus Creator1/8  "R1dC1V"
  R1dC0V/1 -> Bus Creator1/7  "R1dC0V"
  L1dC1V/1 -> Bus Creator1/4  "L1dC1V"
  L1dC0V/1 -> Bus Creator1/3  "L1dC0V"
  L1dC3V/1 -> Bus Creator1/6  "L1dC3V"
  L1dC2V/1 -> Bus Creator1/5  "L1dC2V"
  R1bIsLineExis/1 -> Bus Creator1/14  "R1bIsLineExis"
  L1bIsLineExist/1 -> Bus Creator1/13  "L1bIsLineExist"
  R1dDisFront/1 -> Bus Creator1/12  "R1dDisFront"
  L1dDisFront/1 -> Bus Creator1/11  "L1dDisFront"
  R1dC3V/1 -> Bus Creator1/10  "R1dC3V"
  R1dC2V/1 -> Bus Creator1/9  "R1dC2V"
  kap/1 -> Bus Creator1/2  "kap"
  velSubj/1 -> Bus Creator1/1  "velSubj"
  VlcInternalAcc/1 -> JerkIC/3(VlcInternalAcc)  "VlcInternalAcc"
  RFM_UpdateCnt/1 -> Bus Creator1/21  "RFM_UpdateCnt"
  tCycle/1 -> Bus Creator1/22  "tCycle"
  AccelArbIC/1(accelIC) -> AccelBandIC/1(accelIC), JerkIC/1(accelIC), [accelIC], accelIC/1  "LongCtrl_accelIC"
  Bus Selector1/1 -> AccelKap/1(velSubj), AccelCurvature/2(velSubj)  "<velSubj>"
  JerkIC/1(upperJerkIC) -> upperJerkIC/1  "LongCtrl_upperJerkIC"
  AccelCurvature/1(accelCurvature) -> AccelArbIC/2(accelCurvature)
  AccelKap/1(accelKap) -> AccelArbIC/3(accelKap)
  Bus Selector1/2 -> AccelKap/2(kap)  "<kap>"
  AccelBandIC/1(upperBandIC) -> upperBandIC/1  "LongCtrl_upperBandIC"
  AccelArbIC/2(IC_state) -> JerkIC/2(IC_state)
  JerkIC/2(LowerJerkIC) -> lowerJerkIC/1  "LongCtrl_lowerJerkIC"
  AccelBandIC/2(lowerBandIC) -> lowerBandIC/1  "LongCtrl_lowerBandIC"
  CurvatureOfRoadCalc/1(CurvatureOfRoad) -> AccelCurvature/1(curvatureForCurveDecel)
  Bus Selector3/2 -> CurvatureOfMapCalc/2(i_road_curvature)  "<i_road_curvature>"
  Bus Selector3/3 -> CurvatureOfMapCalc/3(i_road_curvature_far)  "<i_road_curvature_far>"
  Bus Selector3/1 -> CurvatureOfMapCalc/1(velSubj)  "<velSubj>"
  Bus Selector3/6 -> CurvatureOfMapCalc/6(i_road_curvature_distance_matrix)  "<i_road_curvature_distance_matrix>"
  Bus Selector3/4 -> CurvatureOfMapCalc/4(i_road_curvature_far_distance)  "<i_road_curvature_far_distance>"
  Bus Selector3/5 -> CurvatureOfMapCalc/5(i_road_curvature_value_matrix)  "<i_road_curvature_value_matrix>"
  CurvatureOfMapCalc/1(accelDesCurvatureMap) -> AccelArbIC/1(accelMap)
  Bus Selector3/7 -> CurvatureOfMapCalc/7(i_road_curvature_matrix_size)  "<i_road_curvature_matrix_size>"

== system PvtSubSys_PLAN_AP/AP/AP/ORD ==
  velOffRampLimit : Inport
  distRamp2Cur : Inport  Port=2
  vehicleSpd : Inport  Port=3
  BandJerkCalc : Subsystem
  ORD : Stateflow chart  TreatAsAtomicUnit=on
  accelORD : Outport
  upperBandORD : Outport  Port=2
  lowerBandORD : Outport  Port=3
  upperJerkORD : Outport  Port=4
  lowerJerkORD : Outport  Port=5
  wires:
  velOffRampLimit/1 -> ORD/2(velOffRampLimit)
  vehicleSpd/1 -> ORD/1(vehicleSpd)
  distRamp2Cur/1 -> ORD/3(distRamp2Cur)
  ORD/1(accelOffRamp) -> accelORD/1, BandJerkCalc/1(accelOffRamp)  "LongCtrl_accelORD"
  BandJerkCalc/4(lowerJerkORD) -> lowerJerkORD/1  "lowerJerkORD"
  BandJerkCalc/1(upperBandORD) -> upperBandORD/1  "upperBandORD"
  BandJerkCalc/2(lowerBandORD) -> lowerBandORD/1  "lowerBandORD"
  BandJerkCalc/3(upperJerkORD) -> upperJerkORD/1  "upperJerkORD"

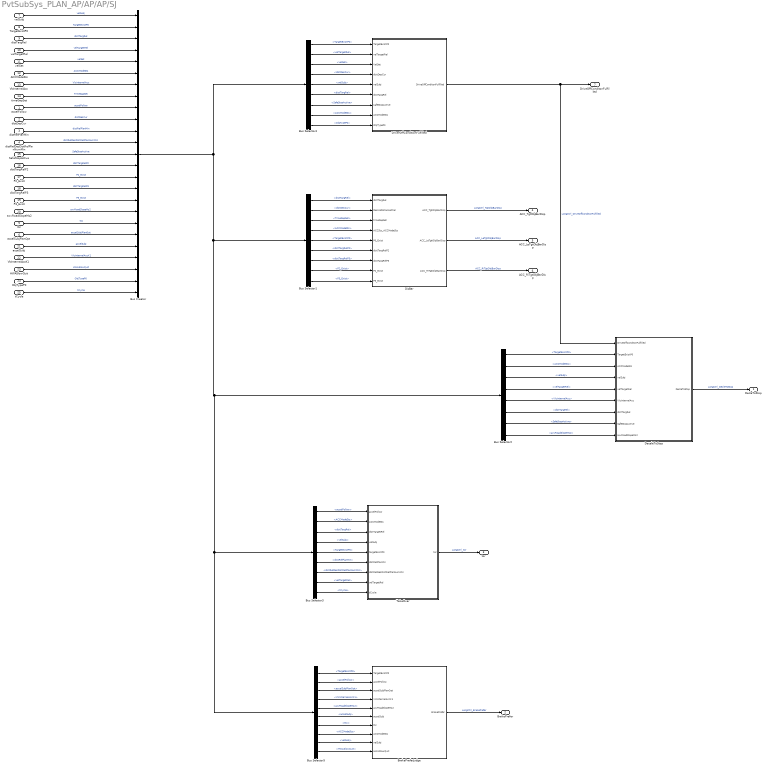
== system PvtSubSys_PLAN_AP/AP/AP/SJ ==
  accelFollow : Inport
  distDesCur : Inport  Port=2
  distRelPlanMin : Inport  Port=3
  distRelDesDistRelPlanNumMin : Inport  Port=4
  ttc : Inport  Port=5
  accelSubjPlanOpt : Inport  Port=6
  velSubj : Inport  Port=7
  TargetExistP0 : Inport  Port=8
  distTargRel : Inport  Port=9
  velTargetRel : Inport  Port=10
  velSet : Inport  Port=11
  ACCModeSts : Inport  Port=12
  VlcInternalAcc : Inport  Port=13
  timeGapSet : Inport  Port=14
  SafeStopActive : Inport  Port=15
  distTargRelP2 : Inport  Port=16
  P2_Exist : Inport  Port=17
  distTargRelP3 : Inport  Port=18
  P3_Exist : Inport  Port=19
  axvRoadSlopeMs2 : Inport  Port=20
  accelSubj : Inport  Port=21
  VlcInternalAccK1 : Inport  Port=22
  HWASlowQuit : Inport  Port=23
  ObjTypeP0 : Inport  Port=24
  tCycle : Inport  Port=25
  BrakePreferJudge : Subsystem
  Bus Creator : BusCreator  Inputs=25
  Bus Selector1 : BusSelector  OutputSignals=distTargRel,distDesCur,TimeGapSet,ACCModeSts,TargetExistP0,distTargRelP2,distTargRelP3,P2_Exist,P3_Exist
  Bus Selector2 : BusSelector  OutputSignals=TargetExistP0,ACCModeSts,velSubj,velTargetRel,VlcInternalAcc,distTargRel,SafeStopActive,axvRoadSlopeMs2
  Bus Selector3 : BusSelector  OutputSignals=accelFollow,ACCModeSts,distTargRel,velSubj,TargetExistP0,distRelPlanMin,distRelDesDistRelPlanNumMin,velTargetRel,tCycle
  Bus Selector4 : BusSelector  OutputSignals=TargetExistP0,velTargetRel,velSet,distDesCur,velSubj,distTargRel,SafeStopActive,ACCModeSts,ObjTypeP0
  Bus Selector5 : BusSelector  OutputSignals=TargetExistP0,accelFollow,accelSubjPlanOpt,VlcInternalAccK1,axvRoadSlopeMs2,accelSubj,ttc,ACCModeSts,velSubj,HWASlowQuit
  DeceleToStop : Subsystem
  DisBar : Subsystem
  DriverOffConditionFulfilled : Subsystem
  TakeOver : Subsystem
  DecleToStop : Outport  OutDataTypeStr=boolean
  BrakePrefer : Outport  Port=2  OutDataTypeStr=boolean
  tor : Outport  Port=3  OutDataTypeStr=boolean
  ACC_TgtObjBarDisp : Outport  Port=4  OutDataTypeStr=uint8
  ACC_LeTgtObjBarDisp : Outport  Port=5  OutDataTypeStr=uint8
  ACC_RiTgtObjBarDisp : Outport  Port=6  OutDataTypeStr=uint8
  DriveOffConditonFulfilled : Outport  Port=7  OutDataTypeStr=boolean
  wires:
  Bus Selector3/9 -> TakeOver/9(tCycle)  "<tCycle>"
  tCycle/1 -> Bus Creator/25  "tCycle"
  Bus Selector4/9 -> DriverOffConditionFulfilled/9(ObjTypeP0)  "<ObjTypeP0>"
  ObjTypeP0/1 -> Bus Creator/24  "ObjTypeP0"
  Bus Selector2/7 -> DeceleToStop/8(SafeStopActive)  "<SafeStopActive>"
  SafeStopActive/1 -> Bus Creator/13  "SafeStopActive"
  Bus Selector3/8 -> TakeOver/8(velTargetRel)  "<velTargetRel>"
  Bus Selector3/7 -> TakeOver/7(distRelDesDistRelPlanNumMin)  "<distRelDesDistRelPlanNumMin>"
  Bus Selector3/6 -> TakeOver/6(distRelPlanMin)  "<distRelPlanMin>"
  distRelDesDistRelPlanNumMin/1 -> Bus Creator/12  "distRelDesDistRelPlanNumMin"
  distRelPlanMin/1 -> Bus Creator/11  "distRelPlanMin"
  Bus Selector3/5 -> TakeOver/5(targetExistP0)  "<TargetExistP0>"
  Bus Selector3/4 -> TakeOver/4(velSubj)  "<velSubj>"
  Bus Selector3/3 -> TakeOver/3(distTargetRel)  "<distTargRel>"
  Bus Selector3/2 -> TakeOver/2(ACCModeSts)  "<ACCModeSts>"
  Bus Selector3/1 -> TakeOver/1(accelFollow)  "<accelFollow>"
  Bus Selector2/1 -> DeceleToStop/2(TargetExistP0)  "<TargetExistP0>"
  Bus Selector2/6 -> DeceleToStop/7(distTargRel)  "<distTargRel>"
  Bus Selector2/2 -> DeceleToStop/3(ACCModeSts)  "<ACCModeSts>"
  Bus Selector2/5 -> DeceleToStop/6(VlcInternalAcc)  "<VlcInternalAcc>"
  Bus Selector2/3 -> DeceleToStop/4(velSubj)  "<velSubj>"
  Bus Selector2/4 -> DeceleToStop/5(velTargetRel)  "<velTargetRel>"
  Bus Selector1/5 -> DisBar/5(P0_Exist)  "<TargetExistP0>"
  Bus Selector1/4 -> DisBar/4(ACCSts_ACCModeSts)  "<ACCModeSts>"
  Bus Selector1/3 -> DisBar/3(timeGapSet)  "<TimeGapSet>"
  Bus Selector1/1 -> DisBar/1(distTargRel)  "<distTargRel>"
  Bus Selector1/2 -> DisBar/2(DesireDistanceChar)  "<distDesCur>"
  Bus Creator/1 -> Bus Selector4/1, Bus Selector1/1, Bus Selector2/1, Bus Selector5/1, Bus Selector3/1
  distDesCur/1 -> Bus Creator/10  "distDesCur"
  accelFollow/1 -> Bus Creator/9  "accelFollow"
  timeGapSet/1 -> Bus Creator/8  "TimeGapSet"
  VlcInternalAcc/1 -> Bus Creator/7  "VlcInternalAcc"
  ACCModeSts/1 -> Bus Creator/6  "ACCModeSts"
  velSet/1 -> Bus Creator/5  "velSet"
  velTargetRel/1 -> Bus Creator/4  "velTargetRel"
  distTargRel/1 -> Bus Creator/3  "distTargRel"
  TargetExistP0/1 -> Bus Creator/2  "TargetExistP0"
  velSubj/1 -> Bus Creator/1  "velSubj"
  TakeOver/1(tor) -> tor/1  "LongCtrl_tor"
  DisBar/1(ACC_TgtObjBarDisp) -> ACC_TgtObjBarDisp/1  "LongCtrl_TgtObjBarDisp"
  DisBar/3(ACC_RiTgtObjBarDisp) -> ACC_RiTgtObjBarDisp/1  "ACC_RiTgtObjBarDisp"
  DisBar/2(ACC_LeTgtObjBarDisp) -> ACC_LeTgtObjBarDisp/1  "ACC_LeTgtObjBarDisp"
  BrakePreferJudge/1(BrakePrefer) -> BrakePrefer/1  "LongCtrl_BrakePrefer"
  DeceleToStop/1(DecleToStop) -> DecleToStop/1  "LongCtrl_DecleToStop"
  DriverOffConditionFulfilled/1(DriveOffConditonFulfilled) -> DriveOffConditonFulfilled/1, DeceleToStop/1(DriveOffConditonFulfilled)  "LongCtrl_DriveOffConditonFulfilled"
  distTargRelP2/1 -> Bus Creator/14  "distTargRelP2"
  P2_Exist/1 -> Bus Creator/15  "P2_Exist"
  distTargRelP3/1 -> Bus Creator/16  "distTargRelP3"
  P3_Exist/1 -> Bus Creator/17  "P3_Exist"
  Bus Selector1/6 -> DisBar/6(distTargRelP2)  "<distTargRelP2>"
  Bus Selector1/7 -> DisBar/7(distTargRelP3)  "<distTargRelP3>"
  Bus Selector1/8 -> DisBar/8(P2_Exist)  "<P2_Exist>"
  Bus Selector1/9 -> DisBar/9(P3_Exist)  "<P3_Exist>"
  axvRoadSlopeMs2/1 -> Bus Creator/18  "axvRoadSlopeMs2"
  Bus Selector2/8 -> DeceleToStop/9(axvRoadSlopeMs2)  "<axvRoadSlopeMs2>"
  Bus Selector4/4 -> DriverOffConditionFulfilled/4(distDesCur)  "<distDesCur>"
  Bus Selector4/2 -> DriverOffConditionFulfilled/2(velTargetRel)  "<velTargetRel>"
  Bus Selector4/5 -> DriverOffConditionFulfilled/5(velSubj)  "<velSubj>"
  Bus Selector4/1 -> DriverOffConditionFulfilled/1(TargetExistP0)  "<TargetExistP0>"
  Bus Selector4/3 -> DriverOffConditionFulfilled/3(VelSet)  "<velSet>"
  Bus Selector4/6 -> DriverOffConditionFulfilled/6(distTargRel)  "<distTargRel>"
  Bus Selector4/7 -> DriverOffConditionFulfilled/7(safeStopActive)  "<SafeStopActive>"
  Bus Selector4/8 -> DriverOffConditionFulfilled/8(ACCModeSts)  "<ACCModeSts>"
  VlcInternalAccK1/1 -> Bus Creator/22  "VlcInternalAccK1"
  accelSubj/1 -> Bus Creator/21  "accelSubj"
  ttc/1 -> Bus Creator/19  "ttc"
  accelSubjPlanOpt/1 -> Bus Creator/20  "accelSubjPlanOpt"
  Bus Selector5/1 -> BrakePreferJudge/1(TargetExistP0)  "<TargetExistP0>"
  Bus Selector5/2 -> BrakePreferJudge/2(accelFollow)  "<accelFollow>"
  Bus Selector5/3 -> BrakePreferJudge/3(accelSubjPlanOpt)  "<accelSubjPlanOpt>"
  Bus Selector5/4 -> BrakePreferJudge/4(VlcInternalAccK1)  "<VlcInternalAccK1>"
  Bus Selector5/5 -> BrakePreferJudge/5(axvRoadSlopeMs2)  "<axvRoadSlopeMs2>"
  Bus Selector5/6 -> BrakePreferJudge/6(accelSubj)  "<accelSubj>"
  Bus Selector5/7 -> BrakePreferJudge/7(ttc)  "<ttc>"
  Bus Selector5/8 -> BrakePreferJudge/8(ACCModeSts)  "<ACCModeSts>"
  Bus Selector5/9 -> BrakePreferJudge/9(velSubj)  "<velSubj>"
  HWASlowQuit/1 -> Bus Creator/23  "HWASlowQuit"
  Bus Selector5/10 -> BrakePreferJudge/10(HWASlowQuit)  "<HWASlowQuit>"

== system PvtSubSys_PLAN_AP/AP/AP/Subsystem ==
  u : Inport
  MATLAB Function : MATLAB Function  TreatAsAtomicUnit=on
  Memory5 : Memory  InheritSampleTime=on
  Tapped Delay2 : simulink/Discrete/Tapped Delay  vinit=0.0  samptime=-1  NumDelays=1  DelayOrder=Newest  includeCurrent=on
  ACCModeSts : Outport
  wires:
  MATLAB Function/1(ACCModeSts) -> ACCModeSts/1
  u/1 -> Tapped Delay2/1
  Tapped Delay2/1 -> MATLAB Function/1(u)
  MATLAB Function/2(CounterK1) -> Memory5/1
  Memory5/1 -> MATLAB Function/2(Counter)

== system PvtSubSys_PLAN_AP/AP/AP/TargetUpdate ==
  TOS_UpdateCnt : Inport
  Detect Change : simulink/Logic and Bit Operations/Detect Change  vinit=0  OutDataTypeStr=boolean
  targUpdate : Outport  OutDataTypeStr=boolean
  wires:
  Detect Change/1 -> targUpdate/1
  TOS_UpdateCnt/1 -> Detect Change/1

== system PvtSubSys_PLAN_AP/AP/AP/VlcInternalAccCalc ==
  VlcInternalAccK1 : Inport
  ACCModeSts : Inport  Port=2  OutDataTypeStr=uint8
  accelSubj : Inport  Port=3
  tCycle : Inport  Port=4
  Chart : Stateflow chart  TreatAsAtomicUnit=on
  Selector1 : Selector  InputPortWidth=19  IndexOptions=Index vector (dialog)  Indices=1  OutputSizes=1
  Tapped Delay : simulink/Discrete/Tapped Delay  vinit=0.0  samptime=-1  NumDelays=1  DelayOrder=Newest  includeCurrent=on
  Tapped Delay1 : simulink/Discrete/Tapped Delay  vinit=0.0  samptime=-1  NumDelays=19  DelayOrder=Oldest  includeCurrent=off
  VlcInternalAccK20 : Outport  OutDataTypeStr=single
  wires:
  Tapped Delay/1 -> Chart/1(ACCModeSts)
  Selector1/1 -> Chart/3(VlcInternalAcc)
  Tapped Delay1/1 -> Selector1/1  "VlcInternalAccK20"
  Chart/1(VlcAcc) -> VlcInternalAccK20/1  "LongCtrl_VlcInternalAccK20"
  tCycle/1 -> Chart/2(tCycle)
  VlcInternalAccK1/1 -> Tapped Delay1/1
  accelSubj/1 -> Chart/4(accelSubj)  "accelSubj"
  ACCModeSts/1 -> Tapped Delay/1

== system PvtSubSys_PLAN_AP/AP/AP/Arbitrate/Subsystem ==
  velPlanEffect : Inport
  velSubjPlanCC : Inport  Port=2
  velSubjPlanFollow : Inport  Port=3
  Constant : Constant  Value=255  OutDataTypeStr=single
  Multiport Switch : MultiPortSwitch  DataPortOrder=Specify indices  DataPortIndices={0,1,2}
  Selector : Selector  InputPortWidth=40  IndexOptions=Index vector (dialog)  Indices=[1:8]  OutputSizes=1
  Signal Conversion : SignalConversion  OverrideOpt=off
  Signal Conversion1 : SignalConversion  OverrideOpt=off
  velSubjPlanArb : Outport
  wires:
  velSubjPlanFollow/1 -> Selector/1
  velPlanEffect/1 -> Multiport Switch/1
  Constant/1 -> Multiport Switch/2
  velSubjPlanCC/1 -> Multiport Switch/3  "LongCtrl_velSubjPlanCC"
  Selector/1 -> Signal Conversion/1
  Multiport Switch/1 -> Signal Conversion1/1
  Signal Conversion/1 -> Multiport Switch/4  "LongCtrl_velSubjPlanFollow"
  Signal Conversion1/1 -> velSubjPlanArb/1  "LongCtrl_velSubjPlanArb"

== system PvtSubSys_PLAN_AP/AP/AP/CCCtrl/AccelCCCalc/CCAcceleNeg ==
  deltaVelCC : Inport  OutDataTypeStr=single  PortDimensions=1
  f : TriggerPort  TriggerType=function-call  VariantControl=Variant
      settings: CopyFcn=Stateflow.SLINSF.SimulinkMan.removeBlockPreDeleteFcn  PreDeleteFcn=Stateflow.SLINSF.SimulinkMan.unsafePredeleteFcn
  1-D Lookup Table : Lookup_n-D  NumberOfTableDimensions=1  BreakpointsForDimension1=P_LongCtrl_CCtAcceleTimeNegCorrXAxis  Table=P_LongCtrl_CCtAcceleTimeNegCorrYAxis  ExtrapMethod=Clip  InternalRulePriority=Speed  RndMeth=Simplest  InputSameDT=on
  P_LongCtrl_CCtAcceleTimeNeg : Constant  Value=P_LongCtrl_CCtAcceleTimeNeg
  Product : Product  Inputs=*/
  Product1 : Product
  accelCC : Outport  OutDataTypeStr=single
  wires:
  Product/1 -> accelCC/1  "CCAccele"
  P_LongCtrl_CCtAcceleTimeNeg/1 -> Product1/1
  deltaVelCC/1 -> 1-D Lookup Table/1, Product/1  "CCDeltaV"
  1-D Lookup Table/1 -> Product1/2
  Product1/1 -> Product/2

== system PvtSubSys_PLAN_AP/AP/AP/CCCtrl/AccelCCCalc/CCAccelePos ==
  deltaVelCC : Inport  OutDataTypeStr=single  PortDimensions=1
  f : TriggerPort  TriggerType=function-call  VariantControl=Variant
      settings: CopyFcn=Stateflow.SLINSF.SimulinkMan.removeBlockPreDeleteFcn  PreDeleteFcn=Stateflow.SLINSF.SimulinkMan.unsafePredeleteFcn
  1-D Lookup Table : Lookup_n-D  NumberOfTableDimensions=1  BreakpointsForDimension1=P_LongCtrl_CCtAcceleTimePosCorrXAxis  Table=P_LongCtrl_CCtAcceleTimePosCorrYAxis  ExtrapMethod=Clip  InternalRulePriority=Speed  RndMeth=Simplest  InputSameDT=on
  P_LongCtrl_CCtAcceleTimePos : Constant  Value=P_LongCtrl_CCtAcceleTimePos
  Product : Product  Inputs=*/
  Product1 : Product
  accelCC : Outport  OutDataTypeStr=single
  wires:
  Product/1 -> accelCC/1  "CCAccele"
  P_LongCtrl_CCtAcceleTimePos/1 -> Product1/1
  deltaVelCC/1 -> 1-D Lookup Table/1, Product/1  "CCDeltaV"
  1-D Lookup Table/1 -> Product1/2
  Product1/1 -> Product/2

== system PvtSubSys_PLAN_AP/AP/AP/CCCtrl/AccelCCCalc/CCDeltaVCalc ==
  CCSetSpd : Inport  OutDataTypeStr=single  PortDimensions=1
  VehicleSpd : Inport  Port=2  OutDataTypeStr=single  PortDimensions=1
  f : TriggerPort  TriggerType=function-call  VariantControl=Variant
      settings: CopyFcn=Stateflow.SLINSF.SimulinkMan.removeBlockPreDeleteFcn  PreDeleteFcn=Stateflow.SLINSF.SimulinkMan.unsafePredeleteFcn
  Add : Sum
  Add1 : Sum  Inputs=+-
  Constant : Constant  Value=3.6  OutDataTypeStr=single
  IPDisVehSpdFac : Constant  Value=P_LongCtrl_CCcoefESPSpd2IPSpd1  OutDataTypeStr=single
  IPDisVehSpdOffset : Constant  Value=P_LongCtrl_CCcoefESPSpd2IPSpd2  OutDataTypeStr=single
  Product : Product
  Product1 : Product  Inputs=*/
  deltaVelCC : Outport
  wires:
  Constant/1 -> Product1/2
  Add1/1 -> Product1/1  "CCDeltaV"
  Product1/1 -> deltaVelCC/1  "CCDeltaV"
  CCSetSpd/1 -> Add1/1  "CCSetSpd"
  Add/1 -> Add1/2
  IPDisVehSpdOffset/1 -> Add/2
  Product/1 -> Add/1
  IPDisVehSpdFac/1 -> Product/2
  VehicleSpd/1 -> Product/1  "VehicleSpd"

== system PvtSubSys_PLAN_AP/AP/AP/CCCtrl/AccelCCCalc/Mph2KphCalc ==
  SpdSetValue : Inport  OutDataTypeStr=single  PortDimensions=1
  f : TriggerPort  TriggerType=function-call  VariantControl=Variant
      settings: CopyFcn=Stateflow.SLINSF.SimulinkMan.removeBlockPreDeleteFcn  PreDeleteFcn=Stateflow.SLINSF.SimulinkMan.unsafePredeleteFcn
  C_LongCtrl_Mph2Kph : Constant  Value=C_LongCtrl_Mph2Kph
  Product : Product
  ACC_SpdSetValueMph2Kph : Outport  OutDataTypeStr=single
  wires:
  Product/1 -> ACC_SpdSetValueMph2Kph/1  "ACC_SpdSetValueMph2Kph"
  C_LongCtrl_Mph2Kph/1 -> Product/2
  SpdSetValue/1 -> Product/1  "SpdSetValue"

== system PvtSubSys_PLAN_AP/AP/AP/CCCtrl/AccelCCLimit ==
  accelCCRaw : Inport
  fastDecel : Inport  Port=2
  IsLaneChange : Inport  Port=3
  SafeStopActive : Inport  Port=4
  Add : Sum  Inputs=+-
  Compare To Constant10 : simulink/Logic and Bit Operations/Compare To Constant  relop=>  const=P_LongCtrl_CCaccelMaxLCActive  OutDataTypeStr=boolean
  Constant : Constant  Value=P_LongCtrl_CCaccelMinFastDecel  OutDataTypeStr=single
  Constant1 : Constant  Value=P_LongCtrl_CCaccelMinNoFastDecel  OutDataTypeStr=single
  Gain : Gain  Gain=50  OutDataTypeStr=single
  Logical Operator2 : Logic  AllPortsSameDT=off  OutDataTypeStr=boolean
  P_LongCtrl_CCaccelLowerIsLaneChange : Constant  Value=P_LongCtrl_CCaccelLowerIsLaneChange  OutDataTypeStr=single
  P_LongCtrl_CCaccelUpperCC : Constant  Value=P_LongCtrl_CCaccelUpperCC  OutDataTypeStr=single
  P_LongCtrl_CCaccelUpperCCSafeStop : Constant  Value=P_LongCtrl_CCaccelUpperCCSafeStop  OutDataTypeStr=single
  Product8 : Product
  SSCaDtIsLaneChange : Constant  Value=0.05  OutDataTypeStr=single
  Saturation Dynamic2 : simulink/Discontinuities/Saturation Dynamic  OutMin=[]  OutMax=[]  OutDataTypeStr=single  OutputDataTypeScalingMode=single  OutDataType=fixdt(1, 16)  OutScaling=2^-10  RndMeth=Nearest  DoSatur=off
  Switch : Switch  Criteria=u2 > Threshold
  Switch1 : Switch  Criteria=u2 > Threshold
  Switch2 : Switch  Criteria=u2 ~= 0
  Switch3 : Switch  Criteria=u2 > Threshold
  TrueDurationTime : TrueDurationTime/TrueDurationTime  TCycle=0.02
  tCycle1 : Constant  Value=0  OutDataTypeStr=single
  accelCCLim : Outport
  wires:
  Switch3/1 -> Saturation Dynamic2/1
  P_LongCtrl_CCaccelUpperCCSafeStop/1 -> Switch3/1
  SafeStopActive/1 -> Switch3/2
  Compare To Constant10/1 -> Logical Operator2/1
  Product8/1 -> Switch2/1
  SSCaDtIsLaneChange/1 -> Product8/1
  Switch1/1 -> Saturation Dynamic2/3
  [LaneChangeCounter] -> Product8/2
  TrueDurationTime/1 -> Gain/1
  Add/1 -> Saturation Dynamic2/2
  accelCCRaw/1 -> Add/1, Compare To Constant10/1
  Logical Operator2/1 -> Switch2/2, Switch1/2, TrueDurationTime/1
  Switch2/1 -> Add/2
  tCycle1/1 -> Switch2/3
  P_LongCtrl_CCaccelUpperCC/1 -> Switch3/3
  Saturation Dynamic2/1 -> accelCCLim/1
  IsLaneChange/1 -> Logical Operator2/2
  Gain/1 -> [LaneChangeCounter]
  P_LongCtrl_CCaccelLowerIsLaneChange/1 -> Switch1/1
  Switch/1 -> Switch1/3
  fastDecel/1 -> Switch/2
  Constant1/1 -> Switch/3
  Constant/1 -> Switch/1

== system PvtSubSys_PLAN_AP/AP/AP/CCCtrl/AcceleBandCC/CCNegAcceleBandCalc ==
  accelCCDes : Inport  OutDataTypeStr=single  PortDimensions=1
  f : TriggerPort  TriggerType=function-call  VariantControl=Variant
      settings: CopyFcn=Stateflow.SLINSF.SimulinkMan.removeBlockPreDeleteFcn  PreDeleteFcn=Stateflow.SLINSF.SimulinkMan.unsafePredeleteFcn
  Add : Sum
  Add1 : Sum
  MinMax : MinMax  Function=max  Inputs=2
  MinMax1 : MinMax  Inputs=2
  P_LongCtrl_CCaMinNegAcceleLowerBand : Constant  Value=P_LongCtrl_CCaMinNegAcceleLowerBand
  P_LongCtrl_CCaMinNegAcceleUpperBand : Constant  Value=P_LongCtrl_CCaMinNegAcceleUpperBand
  P_LongCtrl_CCfacNegAcceleLowerBand : Constant  Value=P_LongCtrl_CCfacNegAcceleLowerBand
  P_LongCtrl_CCfacNegAcceleUpperBand : Constant  Value=P_LongCtrl_CCfacNegAcceleUpperBand
  Product : Product
  Product1 : Product
  accelCCDes1 : InportShadow  OutDataTypeStr=single  PortDimensions=1
  accelCCDes2 : InportShadow  OutDataTypeStr=single  PortDimensions=1
  upperBandCC : Outport  OutDataTypeStr=single
  lowerBandCC : Outport  Port=2  OutDataTypeStr=single
  wires:
  Add1/1 -> MinMax1/2
  accelCCDes2/1 -> Add1/2  "accelCCDes"
  Add/1 -> MinMax/1
  accelCCDes1/1 -> Add/2  "accelCCDes"
  MinMax1/1 -> lowerBandCC/1  "lowerBandCC"
  MinMax/1 -> upperBandCC/1  "upperBandCC"
  Product1/1 -> MinMax1/1
  P_LongCtrl_CCaMinNegAcceleLowerBand/1 -> Add1/1
  P_LongCtrl_CCfacNegAcceleLowerBand/1 -> Product1/2
  P_LongCtrl_CCaMinNegAcceleUpperBand/1 -> Add/1
  Product/1 -> MinMax/2
  P_LongCtrl_CCfacNegAcceleUpperBand/1 -> Product/1
  accelCCDes/1 -> Product/2, Product1/1  "accelCCDes"

== system PvtSubSys_PLAN_AP/AP/AP/CCCtrl/AcceleBandCC/CCPosAcceleBandCalc ==
  accelCCDes : Inport  OutDataTypeStr=single  PortDimensions=1
  f : TriggerPort  TriggerType=function-call  VariantControl=Variant
      settings: CopyFcn=Stateflow.SLINSF.SimulinkMan.removeBlockPreDeleteFcn  PreDeleteFcn=Stateflow.SLINSF.SimulinkMan.unsafePredeleteFcn
  Add : Sum
  Add1 : Sum
  MinMax : MinMax  Function=max  Inputs=2
  MinMax1 : MinMax  Inputs=2
  P_LongCtrl_CCaMinPosAcceleLowerBand : Constant  Value=P_LongCtrl_CCaMinPosAcceleLowerBand
  P_LongCtrl_CCaMinPosAcceleUpperBand : Constant  Value=P_LongCtrl_CCaMinPosAcceleUpperBand
  P_LongCtrl_CCfacPosAcceleLowerBand : Constant  Value=P_LongCtrl_CCfacPosAcceleLowerBand
  P_LongCtrl_CCfacPosAcceleUpperBand : Constant  Value=P_LongCtrl_CCfacPosAcceleUpperBand
  Product : Product
  Product1 : Product
  accelCCDes1 : InportShadow  OutDataTypeStr=single  PortDimensions=1
  accelCCDes2 : InportShadow  OutDataTypeStr=single  PortDimensions=1
  upperBandCC : Outport  OutDataTypeStr=single
  lowerBandCC : Outport  Port=2  OutDataTypeStr=single
  wires:
  Add1/1 -> MinMax1/2
  accelCCDes2/1 -> Add1/2  "accelCCDes"
  Add/1 -> MinMax/1
  accelCCDes1/1 -> Add/2  "accelCCDes"
  MinMax1/1 -> lowerBandCC/1  "lowerBandCC"
  MinMax/1 -> upperBandCC/1  "upperBandCC"
  Product1/1 -> MinMax1/1
  P_LongCtrl_CCaMinPosAcceleLowerBand/1 -> Add1/1
  P_LongCtrl_CCfacPosAcceleLowerBand/1 -> Product1/2
  P_LongCtrl_CCaMinPosAcceleUpperBand/1 -> Add/1
  Product/1 -> MinMax/2
  P_LongCtrl_CCfacPosAcceleUpperBand/1 -> Product/1
  accelCCDes/1 -> Product/2, Product1/1  "accelCCDes"
